simulink model "sampleModel217"  (R2021b)
settings: Solver=VariableStepAuto  StartTime=0.0  StopTime=10.0  RelTol=1e-3
undefined symbols (not defined in the file or in its folder): Newton, Raphson
libraries: simulink x9, slpidlib x1
settings Model: Creator=user  LastModifiedBy=user

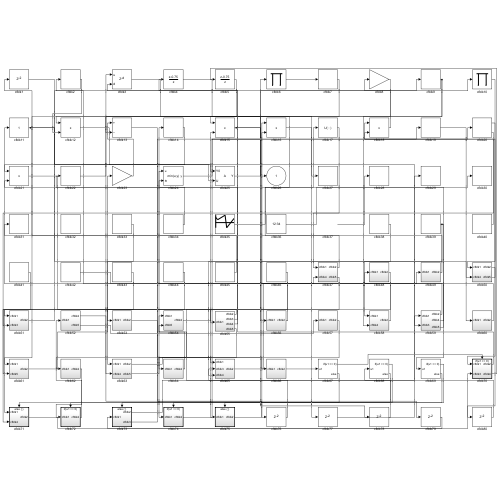
[thumbnail: Simulink's stored preview of the top-level diagram]
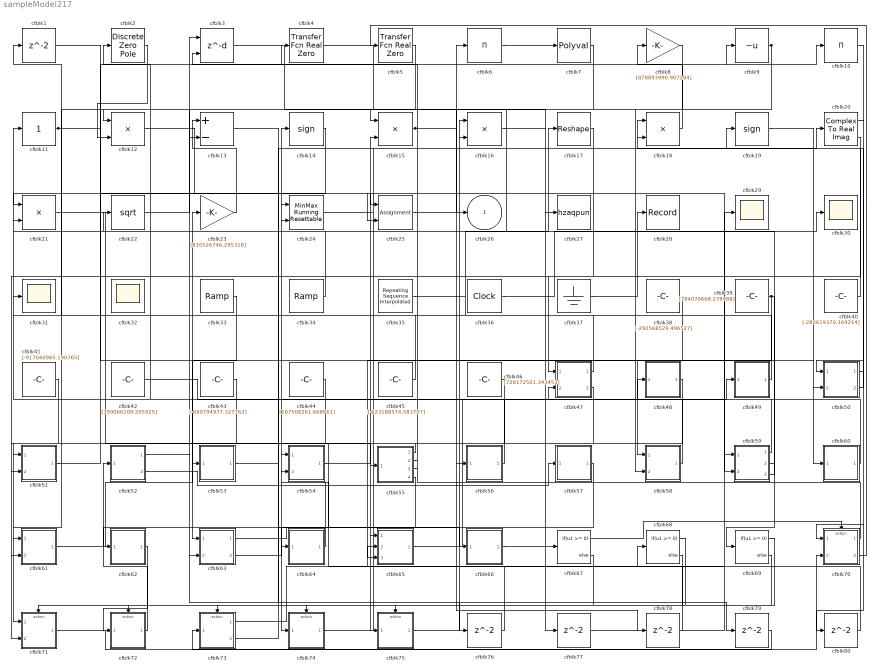
== system sampleModel217 ==
  cfblk{1,76..80} (6 alike) : Delay  SampleTime=1
  cfblk10 : Product  Inputs=*
  cfblk11 : simulink/Math Operations/Slider Gain  gain=1  low=0  high=2
  cfblk12 : Product  Inputs=**
  cfblk13 : Sum  Inputs=+-
  cfblk14 : Signum
  cfblk15 : Product
  cfblk16 : Product
  cfblk17 : Reshape
  cfblk18 : Product  Inputs=**
  cfblk19 : Signum
  cfblk2 : DiscreteZeroPole  Poles=[0 0.5]  Gain=1
  cfblk20 : ComplexToRealImag
  cfblk21 : Product
  cfblk22 : Sqrt  SaturateOnIntegerOverflow=on
  cfblk23 : Gain  Gain=[810526746.295318]
  cfblk24 : simulink/Math Operations/MinMax Running Resettable  Function=min  vinit=0.0
  cfblk25 : Assignment  DiagnosticForDimensions=Warning  IndexOptions=Index vector (dialog)  Indices=1  OutputSizes=1
  cfblk27 : ToWorkspace  VariableName=hzaqpun  SaveFormat=Timeseries  SampleTime=-1
  cfblk28 : Record  FileSettingsInternal="{\"entries\":[{\"content\":{\"excelSettings\":{\"content\":{},\"type\":\"Streamout.ExcelSettings\"}},\"type\":\"Streamout.FileSettingStorage\",\"uuid\":\"24ff093a-1f23-429e-a84e-9bae867bdd3c\"}],\"packageUris\":[\"http://schema.mathworks.com/mf0/streamout_blocks/R2020a\"],\"version\":\"1.0\"}"  SignalsInternal="{\"entries\":[{\"content\":{\"signals\":[{\"content\":{\"blockPath\":[\"sampleModel217/cfblk28\"],\"channel\":[],\"dimensions\":[1],\"domain\":\"sampleModel217/cfblk28\",\"lineColor\":\"#a2142f\",\"plots\":[1],\"port\":1,\"sid\":[\"\"],\"signalID\":8365,\"signalName\":\"cfblk37\"},\"type\":\"RecordBlkView.Signal\",\"uuid\":\"3e2e97f5-1a37-4873-8e35-5f65989afa2d\"}]},\"type\":\"RecordBlkView.InputSignals\",\"uuid\":\"f65d37d0-2da0-4d1a-9cf4-d7ef2a7cb282\"}],\"packageUris\":[\"http://schema.mathworks.com/mf0/streamout_blocks/R2020a\"],\"version\":\"1.0\"}"  VisualizationBindings="{\"sparklinesplugin\":{\"info\":[{\"bindingParametersList\":[],\"subplotID\":1}]}}"
  cfblk{29..32} (4 alike) : Scope
      cfblk32 settings: Floating=on
  cfblk3 : Delay  DelayLengthSource=Input port  SampleTime=1
      settings: InputPortMap=u0,p1
  cfblk33 : simulink/Sources/Ramp  slope=[495.255422]  start=[31.468128]  InitialOutput=[-2500.588137]
  cfblk34 : simulink/Sources/Ramp  slope=[-8058.148753]  start=[37.650933]  InitialOutput=[-350565.854488]
  cfblk35 : simulink/Sources/Repeating Sequence Interpolated  OutValues=[406518574.679400, 231792619.553993, 579583340.287631, -405971187.986971, 321868774.576845]  TimeValues=[0 0.1 0.5 0.6 1].'  LookUpMeth=Interpolation-Use End Values  tsamp=0.01  OutMin=[]  OutMax=[]  OutDataTypeStr=double  OutputDataTypeScalingMode=double  OutDataType=fixdt(0,8)  OutScaling=2^-10
  cfblk36 : DigitalClock
  cfblk37 : Ground
  cfblk38 : Constant  Value=[-292568529.496527]  SampleTime=1
  cfblk39 : Constant  Value=[784070668.278988]  SampleTime=1
  cfblk4 : simulink/Discrete/Transfer Fcn Real Zero  ZeroZ=0.75  ICPrevInput=0.0  DoSatur=off
      settings: SourceProductBaseCode=SL
  cfblk40 : Constant  Value=[-282619370.169214]  SampleTime=1
  cfblk41 : Constant  Value=[-917040985.190765]  SampleTime=1
  cfblk42 : Constant  Value=[399060109.205925]  SampleTime=1
  cfblk43 : Constant  Value=[-660794977.327763]  SampleTime=1
  cfblk44 : Constant  Value=[187508261.668661]  SampleTime=1
  cfblk45 : Constant  Value=[-623188574.583707]  SampleTime=1
  cfblk46 : Constant  Value=[728172501.343453]  SampleTime=1
  cfblk47 : Subsystem
  cfblk48 : Subsystem
  cfblk49 : Subsystem
  cfblk5 : simulink/Discrete/Transfer Fcn Real Zero  ZeroZ=0.75  ICPrevInput=0.0  DoSatur=off
      settings: SourceProductBaseCode=SL
  cfblk50 : Subsystem
  cfblk51 : Subsystem
  cfblk52 : Subsystem
  cfblk53 : Subsystem
  cfblk54 : Subsystem
  cfblk55 : Subsystem
  cfblk56 : Subsystem
  cfblk57 : Subsystem
  cfblk58 : Subsystem
  cfblk59 : Subsystem
  cfblk6 : Product  Inputs=*
  cfblk60 : Subsystem
  cfblk61 : Subsystem
  cfblk62 : Subsystem
  cfblk63 : Subsystem
  cfblk64 : Subsystem
  cfblk65 : Subsystem
  cfblk66 : Subsystem
  cfblk67 : If  IfExpression=u1 >= 0  SampleTime=1
  cfblk68 : If  IfExpression=u1 >= 0  SampleTime=1
  cfblk69 : If  IfExpression=u1 >= 0  SampleTime=1
  cfblk7 : Polyval  Coefs=[ +2.081618890e-019, -1.441693666e-014, +4.719686976e-010, -8.536869453e-006, +1.621573104e-001, -8.087801117e+001 ]
  cfblk70 : Subsystem  TreatAsAtomicUnit=on
  cfblk71 : Subsystem  TreatAsAtomicUnit=on
  cfblk72 : Subsystem  TreatAsAtomicUnit=on
  cfblk73 : Subsystem  TreatAsAtomicUnit=on
  cfblk74 : Subsystem  TreatAsAtomicUnit=on
  cfblk75 : Subsystem  TreatAsAtomicUnit=on
  cfblk8 : Gain  Gain=[878893990.907284]
  cfblk9 : UnaryMinus
  cfblk26 : Outport
  wires:
  cfblk6/1 -> cfblk7/1
  cfblk36/1 -> cfblk30/1
  cfblk59/1(cfblk2) -> cfblk16/1
  cfblk57/1(cfblk2) -> cfblk74/1(cfblk1)
  cfblk50/1(cfblk2) -> cfblk70/1(cfblk1)
  cfblk34/1 -> cfblk14/1
  cfblk45/1 -> cfblk11/1
  cfblk49/1(cfblk2) -> cfblk12/1
  cfblk65/1(cfblk2) -> cfblk49/1(cfblk1)
  cfblk33/1 -> cfblk63/1(cfblk1)
  cfblk2/1 -> cfblk12/2
  cfblk17/1 -> cfblk47/1(cfblk1)
  cfblk8/1 -> cfblk15/1
  cfblk39/1 -> cfblk69/1, cfblk65/3(cfblk4)
  cfblk64/1(cfblk2) -> cfblk24/1
  cfblk58/1(cfblk2) -> cfblk2/1
  cfblk43/1 -> cfblk71/1(cfblk1)
  cfblk7/1 -> cfblk51/1(cfblk1)
  cfblk56/1(cfblk2) -> cfblk31/1
  cfblk42/1 -> cfblk47/2(cfblk4)
  cfblk75/1(cfblk2) -> cfblk16/2
  cfblk72/1(cfblk2) -> cfblk52/1(cfblk1)
  cfblk15/1 -> cfblk26/1, cfblk78/1
  cfblk41/1 -> cfblk71/2(cfblk4)
  cfblk20/2 -> cfblk51/2(cfblk3)
  cfblk18/1 -> cfblk8/1
  cfblk52/2(cfblk5) -> cfblk57/1(cfblk1)
  cfblk40/1 -> cfblk18/1
  cfblk24/1 -> cfblk6/1
  cfblk14/1 -> cfblk21/1
  cfblk19/1 -> cfblk60/1(cfblk1)
  cfblk35/1 -> cfblk17/1
  cfblk16/1 -> cfblk27/1
  cfblk10/1 -> cfblk50/1(cfblk1)
  cfblk71/1(cfblk2) -> cfblk70/2(cfblk3)
  cfblk25/1 -> cfblk9/1
  cfblk61/1(cfblk2) -> cfblk23/1
  cfblk55/1(cfblk2) -> cfblk53/1(cfblk1)
  cfblk74/1(cfblk2) -> cfblk20/1
  cfblk46/1 -> cfblk75/1(cfblk1)
  cfblk37/1 -> cfblk28/1
  cfblk5/1 -> cfblk63/2(cfblk4)
  cfblk73/1(cfblk2) -> cfblk29/1
  cfblk60/1(cfblk2) -> cfblk24/2
  cfblk11/1 -> cfblk50/2(cfblk4), cfblk25/2
  cfblk50/2(cfblk5) -> cfblk18/2
  cfblk51/1(cfblk2) -> cfblk10/1
  cfblk62/1(cfblk2) -> cfblk72/1(cfblk1)
  cfblk54/1(cfblk2) -> cfblk15/2
  cfblk63/1(cfblk2) -> cfblk66/1(cfblk1)
  cfblk3/1 -> cfblk56/1(cfblk1)
  cfblk55/2(cfblk3) -> cfblk4/1
  cfblk38/1 -> cfblk58/1(cfblk1)
  cfblk21/1 -> cfblk55/1(cfblk1)
  cfblk12/1 -> cfblk59/2(cfblk3)
  cfblk63/2(cfblk5) -> cfblk54/1(cfblk1)
  cfblk73/2(cfblk3) -> cfblk19/1
  cfblk47/1(cfblk2) -> cfblk1/1
  cfblk48/1(cfblk2) -> cfblk64/1(cfblk1)
  cfblk47/2(cfblk5) -> cfblk61/1(cfblk1)
  cfblk44/1 -> cfblk61/2(cfblk5)
  cfblk23/1 -> cfblk13/1
  cfblk4/1 -> cfblk67/1
  cfblk22/1 -> cfblk3/1
  cfblk13/1 -> cfblk65/1(cfblk1)
  cfblk9/1 -> cfblk13/2, cfblk58/2(cfblk4)
  cfblk59/2(cfblk4) -> cfblk21/2
  cfblk1/1 -> cfblk25/1
  cfblk59/3(cfblk5) -> cfblk48/1(cfblk1)
  cfblk70/1(cfblk2) -> cfblk3/2
  cfblk55/3(cfblk4) -> cfblk22/1
  cfblk55/4(cfblk5) -> cfblk62/1(cfblk1)
  cfblk70/2(cfblk4) -> cfblk5/1
  cfblk67/1 -> cfblk70/Action
  cfblk67/2 -> cfblk71/Action
  cfblk68/1 -> cfblk72/Action
  cfblk68/2 -> cfblk73/Action
  cfblk69/1 -> cfblk74/Action
  cfblk69/2 -> cfblk75/Action
  cfblk53/1(cfblk2) -> cfblk76/1
  cfblk76/1 -> cfblk65/2(cfblk3)
  cfblk66/1(cfblk2) -> cfblk77/1
  cfblk77/1 -> cfblk59/1(cfblk1)
  cfblk78/1 -> cfblk54/2(cfblk5)
  cfblk52/1(cfblk2) -> cfblk79/1
  cfblk79/1 -> cfblk73/1(cfblk1)
  cfblk20/1 -> cfblk80/1
  cfblk80/1 -> cfblk68/1

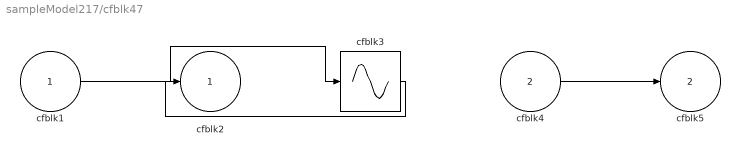
== system sampleModel217/cfblk47 ==
  cfblk1 : Inport
  cfblk4 : Inport  Port=2
  cfblk3 : Sin  TimeSource=Use external signal  SampleTime=0
  cfblk2 : Outport
  cfblk5 : Outport  Port=2
  wires:
  cfblk1/1 -> cfblk3/1
  cfblk4/1 -> cfblk5/1
  cfblk3/1 -> cfblk2/1

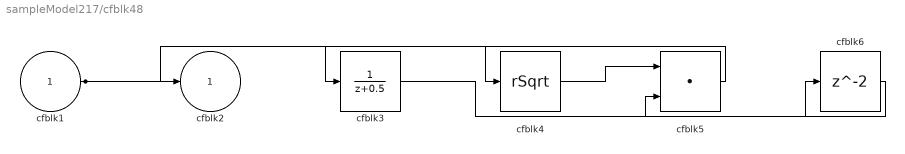
== system sampleModel217/cfblk48 ==
  cfblk1 : Inport
  cfblk3 : DiscreteTransferFcn  SampleTime=1
  cfblk4 : Sqrt  Operator=rSqrt  AlgorithmType=Newton-Raphson  SaturateOnIntegerOverflow=on
  cfblk5 : DotProduct  InputSameDT=on  OutDataTypeStr=Inherit: Inherit via internal rule
  cfblk6 : Delay  SampleTime=1
  cfblk2 : Outport
  wires:
  cfblk4/1 -> cfblk5/1
  cfblk1/1 -> cfblk2/1, cfblk4/1
  cfblk5/1 -> cfblk3/1
  cfblk3/1 -> cfblk6/1
  cfblk6/1 -> cfblk5/2

== system sampleModel217/cfblk49 ==
  cfblk1 : Inport
  cfblk3 : Squeeze
  cfblk4 : simulink/Math Operations/MinMax Running Resettable  Function=min  vinit=0.0
  cfblk2 : Outport
  wires:
  cfblk3/1 -> cfblk2/1, cfblk4/2
  cfblk1/1 -> cfblk3/1, cfblk4/1

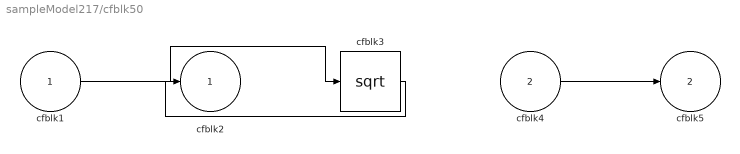
== system sampleModel217/cfblk50 ==
  cfblk1 : Inport
  cfblk4 : Inport  Port=2
  cfblk3 : Sqrt  SaturateOnIntegerOverflow=on
  cfblk2 : Outport
  cfblk5 : Outport  Port=2
  wires:
  cfblk4/1 -> cfblk5/1
  cfblk1/1 -> cfblk3/1
  cfblk3/1 -> cfblk2/1

== system sampleModel217/cfblk51 ==
  cfblk1 : Inport
  cfblk3 : Inport  Port=2
  cfblk2 : Outport
  wires:
  cfblk3/1 -> cfblk2/1

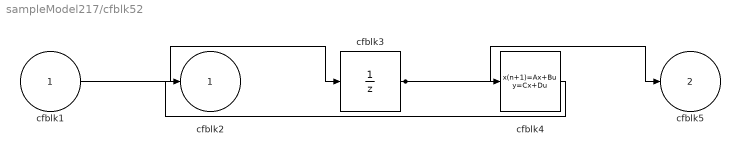
== system sampleModel217/cfblk52 ==
  cfblk1 : Inport
  cfblk3 : UnitDelay  HasFrameUpgradeWarning=on
  cfblk4 : DiscreteStateSpace
  cfblk2 : Outport
  cfblk5 : Outport  Port=2
  wires:
  cfblk1/1 -> cfblk3/1
  cfblk4/1 -> cfblk2/1
  cfblk3/1 -> cfblk5/1, cfblk4/1

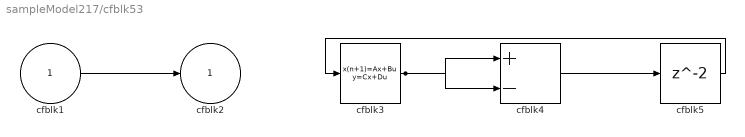
== system sampleModel217/cfblk53 ==
  cfblk1 : Inport
  cfblk3 : DiscreteStateSpace
  cfblk4 : Sum  Inputs=+-
  cfblk5 : Delay  SampleTime=1
  cfblk2 : Outport
  wires:
  cfblk1/1 -> cfblk2/1
  cfblk3/1 -> cfblk4/1, cfblk4/2
  cfblk4/1 -> cfblk5/1
  cfblk5/1 -> cfblk3/1

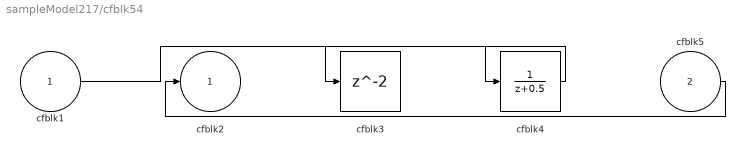
== system sampleModel217/cfblk54 ==
  cfblk1 : Inport
  cfblk5 : Inport  Port=2
  cfblk3 : Delay  SampleTime=1
  cfblk4 : DiscreteTransferFcn  SampleTime=1
  cfblk2 : Outport
  wires:
  cfblk4/1 -> cfblk3/1
  cfblk5/1 -> cfblk2/1
  cfblk1/1 -> cfblk4/1

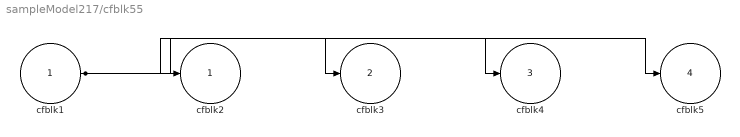
== system sampleModel217/cfblk55 ==
  cfblk1 : Inport
  cfblk2 : Outport
  cfblk3 : Outport  Port=2
  cfblk4 : Outport  Port=3
  cfblk5 : Outport  Port=4
  wires:
  cfblk1/1 -> cfblk5/1, cfblk4/1, cfblk2/1, cfblk3/1

== system sampleModel217/cfblk56 ==
  cfblk1 : Inport
  cfblk3 : Sqrt  SaturateOnIntegerOverflow=on
  cfblk2 : Outport
  wires:
  cfblk1/1 -> cfblk3/1
  cfblk3/1 -> cfblk2/1

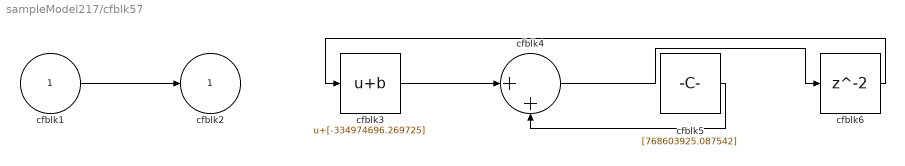
== system sampleModel217/cfblk57 ==
  cfblk1 : Inport
  cfblk3 : Bias  Bias=[-334974696.269725]
  cfblk4 : Sum  Inputs=|++
  cfblk5 : Constant  Value=[768603925.087542]  SampleTime=1
  cfblk6 : Delay  SampleTime=1
  cfblk2 : Outport
  wires:
  cfblk3/1 -> cfblk4/1
  cfblk5/1 -> cfblk4/2
  cfblk1/1 -> cfblk2/1
  cfblk4/1 -> cfblk6/1
  cfblk6/1 -> cfblk3/1

== system sampleModel217/cfblk58 ==
  cfblk1 : Inport
  cfblk4 : Inport  Port=2
  cfblk3 : Constant  Value=[-494485408.007506]  SampleTime=1
  cfblk2 : Outport
  wires:
  cfblk3/1 -> cfblk2/1

== system sampleModel217/cfblk59 ==
  cfblk1 : Inport
  cfblk3 : Inport  Port=2
  cfblk2 : Outport
  cfblk4 : Outport  Port=2
  cfblk5 : Outport  Port=3
  wires:
  cfblk1/1 -> cfblk5/1
  cfblk3/1 -> cfblk4/1, cfblk2/1

== system sampleModel217/cfblk60 ==
  cfblk1 : Inport
  cfblk3 : DiscreteFilter  SampleTime=1
  cfblk4 : Math  Operator=10^u  SaturateOnIntegerOverflow=on
  cfblk2 : Outport
  wires:
  cfblk1/1 -> cfblk4/1
  cfblk3/1 -> cfblk2/1
  cfblk4/1 -> cfblk3/1

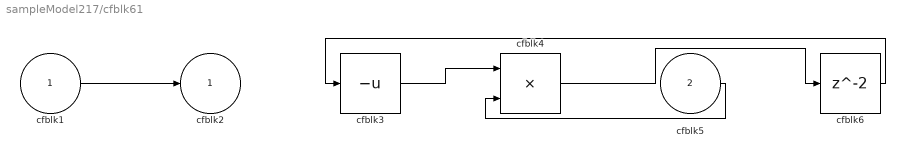
== system sampleModel217/cfblk61 ==
  cfblk1 : Inport
  cfblk5 : Inport  Port=2
  cfblk3 : UnaryMinus
  cfblk4 : Product  Inputs=**
  cfblk6 : Delay  SampleTime=1
  cfblk2 : Outport
  wires:
  cfblk1/1 -> cfblk2/1
  cfblk3/1 -> cfblk4/1
  cfblk5/1 -> cfblk4/2
  cfblk4/1 -> cfblk6/1
  cfblk6/1 -> cfblk3/1

== system sampleModel217/cfblk62 ==
  cfblk1 : Inport
  cfblk3 : Abs
  cfblk2 : Outport
  wires:
  cfblk1/1 -> cfblk3/1
  cfblk3/1 -> cfblk2/1

== system sampleModel217/cfblk63 ==
  cfblk1 : Inport
  cfblk4 : Inport  Port=2
  cfblk3 : Sum  Inputs=+
  cfblk2 : Outport
  cfblk5 : Outport  Port=2
  wires:
  cfblk1/1 -> cfblk5/1
  cfblk3/1 -> cfblk2/1
  cfblk4/1 -> cfblk3/1

== system sampleModel217/cfblk64 ==
  cfblk1 : Inport
  cfblk3 : UnitDelay  HasFrameUpgradeWarning=on
  cfblk2 : Outport
  wires:
  cfblk1/1 -> cfblk3/1
  cfblk3/1 -> cfblk2/1

== system sampleModel217/cfblk65 ==
  cfblk1 : Inport
  cfblk3 : Inport  Port=2
  cfblk4 : Inport  Port=3
  cfblk2 : Outport
  wires:
  cfblk1/1 -> cfblk2/1

== system sampleModel217/cfblk66 ==
  cfblk1 : Inport
  cfblk3 : Sum  Inputs=+-
  cfblk2 : Outport
  wires:
  cfblk3/1 -> cfblk2/1
  cfblk1/1 -> cfblk3/1, cfblk3/2

== system sampleModel217/cfblk70 ==
  cfblk1 : Inport
  cfblk3 : Inport  Port=2
  Action Port : ActionPort  ActionPortLabel=if(u1 >= 0)
  cfblk2 : Outport
  cfblk4 : Outport  Port=2
  wires:
  cfblk1/1 -> cfblk2/1
  cfblk3/1 -> cfblk4/1

== system sampleModel217/cfblk71 ==
  cfblk1 : Inport
  cfblk4 : Inport  Port=2
  Action Port : ActionPort  ActionPortLabel=else
  cfblk3 : Trigonometry
  cfblk2 : Outport
  wires:
  cfblk3/1 -> cfblk2/1
  cfblk1/1 -> cfblk3/1

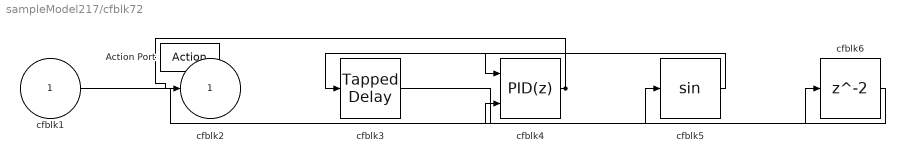
== system sampleModel217/cfblk72 ==
  cfblk1 : Inport
  Action Port : ActionPort  ActionPortLabel=if(u1 >= 0)
  cfblk3 : simulink/Discrete/Tapped Delay  vinit=0.0  samptime=-1  NumDelays=1  DelayOrder=Oldest  includeCurrent=off
  cfblk4 : slpidlib/PID Controller (2DOF)  Controller=PID  Form=Parallel  TimeDomain=Discrete-time  UseExternalTs=off  SampleTime=-1  IntegratorMethod=Forward Euler  FilterMethod=Forward Euler  ControllerParametersSource=internal  P=1  I=1  D=0  UseFilter=on  N=100  b=1  c=1  TunerSelectOption=Transfer Function Based (PID Tuner App)  InitialConditionSource=internal  InitialConditionForIntegrator=0  InitialConditionForFilter=0  DifferentiatorICPrevScaledInput=0  ExternalReset=none  TrackingMode=off  Kt=1  LimitOutput=off  SatLimitsSource=internal  UpperSaturationLimit=inf  LowerSaturationLimit=-inf  LinearizeAsGain=off  AntiWindupMode=none  Kb=1  POutMin=[]  POutMax=[]  IOutMin=[]  IOutMax=[]  DOutMin=[]  DOutMax=[]  NOutMin=[]  NOutMax=[]  bOutMin=[]  bOutMax=[]  cOutMin=[]  cOutMax=[]  SumOutMin=[]  SumOutMax=[]  SaturationOutMin=[]  SaturationOutMax=[]  PParamMin=[]  PParamMax=[]  IParamMin=[]  IParamMax=[]  DParamMin=[]  DParamMax=[]  NParamMin=[]  NParamMax=[]  bParamMin=[]  bParamMax=[]  cParamMin=[]  cParamMax=[]  KbParamMin=[]  KbParamMax=[]  KtParamMin=[]  KtParamMax=[]  KbOutMin=[]  KbOutMax=[]  KtOutMin=[]  KtOutMax=[]  IntegratorOutMin=[]  IntegratorOutMax=[]  FilterOutMin=[]  FilterOutMax=[]  SumI1OutMin=[]  SumI1OutMax=[]  SumI2OutMin=[]  SumI2OutMax=[]  SumI3OutMin=[]  SumI3OutMax=[]  SumI4OutMin=[]  SumI4OutMax=[]  SumDOutMin=[]  SumDOutMax=[]  Sum1OutMin=[]  Sum1OutMax=[]  Sum2OutMin=[]  Sum2OutMax=[]  Sum3OutMin=[]  Sum3OutMax=[]  DifferentiatorOutMin=[]  DifferentiatorOutMax=[]  FilterDiffOutCoefMin=[]  FilterDiffOutCoefMax=[]  ReciprocalOutMin=[]  ReciprocalOutMax=[]  SumDenOutMin=[]  SumDenOutMax=[]  SumNumOutMin=[]  SumNumOutMax=[]  DivideOutMin=[]  DivideOutMax=[]  UdiffTsProdOutMin=[]  UdiffTsProdOutMax=[]  NTsProdOutMin=[]  NTsProdOutMax=[]  UintegralTsProdOutMin=[]  UintegralTsProdOutMax=[]  UngainTsProdOutMin=[]  UngainTsProdOutMax=[]  IntegratorContinuousStateAttributes=''  IntegratorStateMustResolveToSignalObject=off  IntegratorRTWStateStorageClass=Auto  FilterContinuousStateAttributes=''  FilterStateMustResolveToSignalObject=off  FilterRTWStateStorageClass=Auto  ParallelPVariant=InternalParameters  IdealPVariant=Disabled  IVariant=InternalParameters  DVariant=InternalParameters  bVariant=InternalParameters  cVariant=InternalParameters  IntegratorVariant=Discrete  SatVariant=Disabled  AWVariant=Passthrough  PCopyVariant=Disabled  TRVariant=Disabled  FdbkBlocksVariant=Forward  IdealPFdbkVariant=Disabled  SatFdbkVariant=Disabled  DerivativeFilterVariant=ForwardEulerFilter  NVariant=InternalParameters  NCopyVariant=Disabled  FilterICVariant=InternalICsFilter  IntegratorICVariant=InternalICs  ExternalResetVariant=Disabled  TRSumVariant=Passthrough  SumFdbkVariant=Disabled  SumVariant=Sum_PID  TsampFilterVariant=InternalTs  TsampNgainVariant=Passthrough  TsampIntegralVariant=Passthrough  ExternalSaturationOutDataTypeStr=Inherit: Same as second input
      settings: SourceProductBaseCode=SL
  cfblk5 : Trigonometry
  cfblk6 : Delay
  cfblk2 : Outport
  wires:
  cfblk1/1 -> cfblk5/1
  cfblk4/1 -> cfblk2/1, cfblk3/1
  cfblk5/1 -> cfblk4/1
  cfblk3/1 -> cfblk6/1
  cfblk6/1 -> cfblk4/2

== system sampleModel217/cfblk73 ==
  cfblk1 : Inport
  Action Port : ActionPort  ActionPortLabel=else
  cfblk2 : Outport
  cfblk3 : Outport  Port=2
  wires:
  cfblk1/1 -> cfblk2/1, cfblk3/1

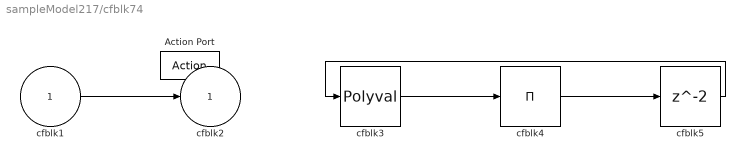
== system sampleModel217/cfblk74 ==
  cfblk1 : Inport
  Action Port : ActionPort  ActionPortLabel=if(u1 >= 0)
  cfblk3 : Polyval  Coefs=[ +2.081618890e-019, -1.441693666e-014, +4.719686976e-010, -8.536869453e-006, +1.621573104e-001, -8.087801117e+001 ]
  cfblk4 : Product  Inputs=*
  cfblk5 : Delay
  cfblk2 : Outport
  wires:
  cfblk3/1 -> cfblk4/1
  cfblk1/1 -> cfblk2/1
  cfblk4/1 -> cfblk5/1
  cfblk5/1 -> cfblk3/1

== system sampleModel217/cfblk75 ==
  cfblk1 : Inport
  Action Port : ActionPort  ActionPortLabel=else
  cfblk3 : Product
  cfblk2 : Outport
  wires:
  cfblk1/1 -> cfblk2/1, cfblk3/1, cfblk3/2
